simulink model "model_closedloop"  (R2019b)
settings: Solver=FixedStepAuto  StartTime=0.0  StopTime=t_end  FixedStep=dt  MaxStep=.1  RelTol=1e-3
undefined symbols (not defined in the file): ref2Pos, Ts, yMask
settings Model: Creator=enrique.babio  LastModifiedBy=enrique.babio
settings DataIOCC: ExternalInput=getinputstruct(opTrim)  InitialState=getstatestruct(opTrim)  SaveState=on

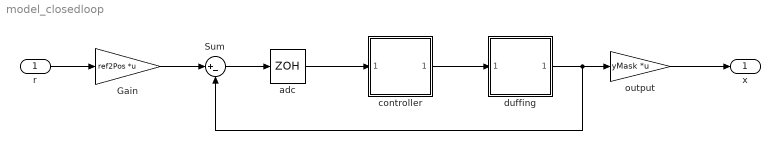
== system model_closedloop ==
  r : Inport
  Gain : Gain  Gain=ref2Pos  Multiplication=Matrix(K*u)
  Sum : Sum  Inputs=|+-
  adc : ZeroOrderHold  SCDEnableBlockLinearizationSpecification=on  SampleTime=Ts
  controller : Subsystem  TreatAsAtomicUnit=on  ReferencedSubsystem=controller
  duffing : Subsystem  ReferencedSubsystem=duffing
  output : Gain  Gain=yMask  Multiplication=Matrix(K*u)
  x : Outport
  wires:
  controller/1 -> duffing/1
  Sum/1 -> adc/1
  duffing/1 -> output/1, Sum/2
  r/1 -> Gain/1
  Gain/1 -> Sum/1
  output/1 -> x/1
  adc/1 -> controller/1
